simulink model "Q5"  (Simulink 7.2)
settings: Solver=ode45  StartTime=0.0  StopTime=200  RelTol=1e-3
undefined symbols (not defined in the file): A, B, C, Kdisc, Ts
settings Model: Creator=Mikkel  LastModifiedBy=Mahler

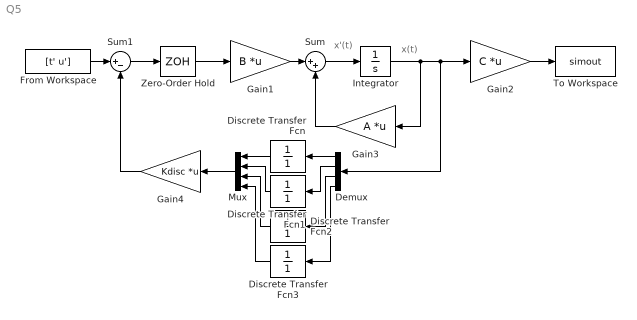
== system Q5 ==
  note: x(t)
  note: x'(t)
  Demux : Demux  Orientation=left
  Discrete Transfer Fcn{,1..3} (4 alike) : DiscreteTransferFcn  Orientation=left  Denominator=[1]  SampleTime=Ts
  From Workspace : FromWorkspace  VariableName=[t' u']  SampleTime=0
  Gain1 : Gain  Gain=B  Multiplication=Matrix(K*u)  ParameterDataType=sfix(16)  ParameterScaling=2^0  OutDataType=sfix(16)  OutScaling=2^0
  Gain2 : Gain  Gain=C  Multiplication=Matrix(K*u)  ParameterDataType=sfix(16)  ParameterScaling=2^0  OutDataType=sfix(16)  OutScaling=2^0
  Gain3 : Gain  Orientation=left  Gain=A  Multiplication=Matrix(K*u)  ParameterDataType=sfix(16)  ParameterScaling=2^0  OutDataType=sfix(16)  OutScaling=2^0
  Gain4 : Gain  Orientation=left  Gain=Kdisc  Multiplication=Matrix(K*u)  ParameterDataType=sfix(16)  ParameterScaling=2^0  OutDataType=sfix(16)  OutScaling=2^0
  Integrator : Integrator
  Mux : Mux  Orientation=left
  Sum : Sum  Inputs=|++  OutDataType=sfix(16)  OutScaling=2^0
  Sum1 : Sum  Inputs=|+-  OutDataType=sfix(16)  OutScaling=2^0
  To Workspace : ToWorkspace  VariableName=simout  SampleTime=-1  SaveFormat=Structure With Time
  Zero-Order Hold : ZeroOrderHold  SampleTime=Ts
  wires:
  Gain1/1 -> Sum/1
  Sum/1 -> Integrator/1
  Integrator/1 -> Gain2/1, Demux/1, Gain3/1
  Gain3/1 -> Sum/2
  Gain2/1 -> To Workspace/1
  Sum1/1 -> Zero-Order Hold/1
  Gain4/1 -> Sum1/2
  From Workspace/1 -> Sum1/1
  Mux/1 -> Gain4/1
  Zero-Order Hold/1 -> Gain1/1
  Demux/1 -> Discrete Transfer Fcn/1
  Discrete Transfer Fcn/1 -> Mux/1
  Demux/2 -> Discrete Transfer Fcn1/1
  Discrete Transfer Fcn1/1 -> Mux/2
  Demux/3 -> Discrete Transfer Fcn2/1
  Discrete Transfer Fcn2/1 -> Mux/3
  Demux/4 -> Discrete Transfer Fcn3/1
  Discrete Transfer Fcn3/1 -> Mux/4
